simulink model "Crane_rigid_3d_single_20_coupling_tracking"  (R2021b)
settings: Solver=ode15s  StartTime=0.0  StopTime=t_f  MaxStep=1e-3  RelTol=1e-3
values from neighbouring files (symbols this model uses):
  h = 1e-5    (= 1e-05)    [Conference_paper.m]    (also in Latest.m)
  m = 10    [Conference_paper.m]    (also in Latest.m = 100; control_8_collocated_PD_tracking.m = load_mass+hook_mass+cable_mass_total)
  N = floor(t_f / h)    [control_2_zero_vibration.m]    (also in control_3_ZVD.m; modify_tracking.m = 3)
  s = c1*(x-xd)+c2*(v-vd)+c3*theta_dot_1+c4*theta_1    [control_10_SMC_single_first_explicit.m]    (also in control_11_SMC_single_first_implicit.m = c1*(x-xd)+c2*(v-vd)+c3*theta_dot+c4*theta; control_12_SMC_single_last_explicit.m = c1*(x-xd)+c2*(v-vd)+c3*theta_dot_2+c4*theta_2; control_13_SMC_single_last_implicit.m = c1*(x-xd)+c2*(v-vd)+c3*theta_dot+c4*theta; control_14_SMC_double_explicit.m = (v-vd)+lambda*(x-xd)+alpha*theta_1+beta*theta_2)
  sin_traj_w = 0.5    [modify_tracking.m]
  X = ex+lambda*sin(theta)    [control_16_PD_energy_first.m]    (also in control_17_PD_energy_last.m)
  Z = cont_param_8(4)    [control_8_collocated_PD_tracking.m]
undefined symbols (not defined in the file or in its folder): all_initial_sway, c_actuator, cable_mass_total, cart_disturbance_amp, cart_mass, delay_time, first_link_sway, hook_mass, load_disturbance_amp, payload_mass, sat_const, sin_traj_A, total_mass, traj_number, Y
libraries: nesl_utility x19, sm_lib x15
settings Model: Creator=rmoja  LastModifiedBy=SESA642626

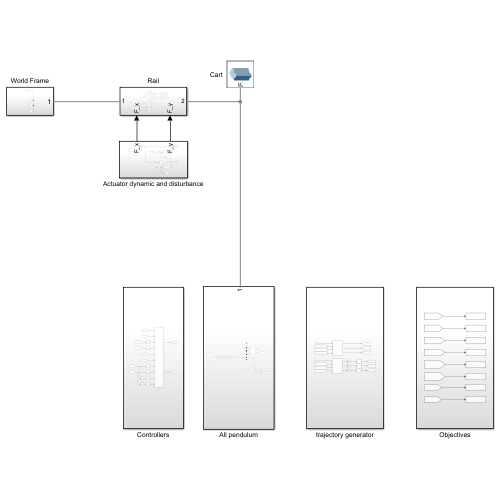
[thumbnail: Simulink's stored preview of the top-level diagram]
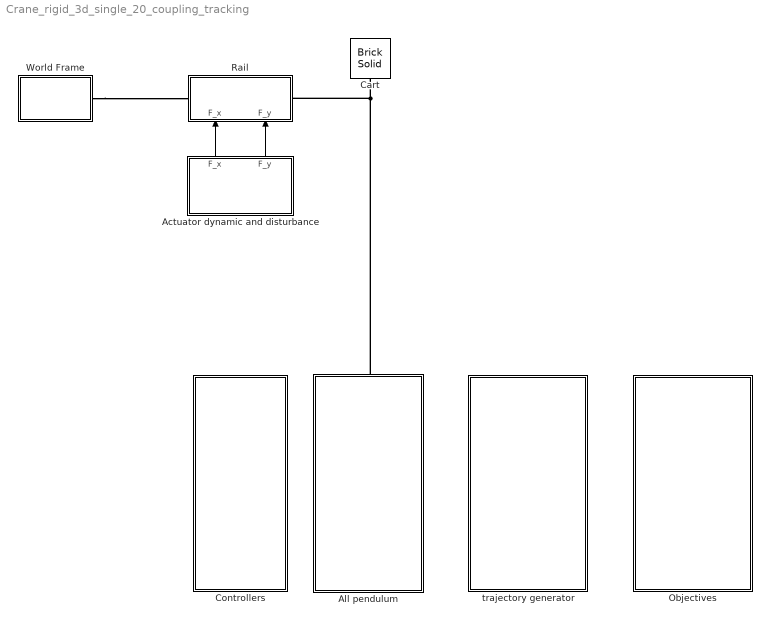
== system Crane_rigid_3d_single_20_coupling_tracking ==
  Actuator dynamic and disturbance : Subsystem
  All pendulum : Subsystem
      settings: PortSchema="{\"entries\":[{\"content\":{\"sides\":[{\"content\":{\"connectorIds\":[]},\"type\":\"ConnectorPlacement.EquallySpacedRectSide\",\"uuid\":\"a0695cec-8b60-4481-8da3-91054655feca\"},{\"content\":{\"connectorIds\":[],\"side\":\"RIGHT\"},\"type\":\"ConnectorPlacement.EquallySpacedRectSide\",\"uuid\":\"63fc90b5-61bb-43b2-b1de-87e85d16d1ba\"},{\"content\":{\"connectorIds\":[\"LConn1\"],\"side\":\"TOP\"},\"type\":\"ConnectorPlacement.EquallySpacedRectSide\",\"uuid\":\"b1a79959-5d9b-4237-a357-9ee6cf3ddb2d\"}]},\"type\":\"ConnectorPlacement.EquallySpacedConnector\",\"uuid\":\"2998d234-7b55-409a-8879-2241677dc568\"}],\"packageUris\":[\"http://schema.mathworks.com/mf0/Connector/R2020b\"],\"version\":\"1.0\"}"
  Cart : sm_lib/Body Elements/Brick Solid  GraphicAmbientColor=[0.15 0.15 0.15 1.0]  BasedOnType=Mass  BrickDimensions=[1 1 1]  BrickDimensionUnits=m  CenterOfMass=[0 0 0]  CenterOfMassUnits=m  GraphicDiffuseColor=[0.8 0.0 0.8]  Density=1000  DensityUnits=kg/(m^3)  DoExposeReferenceFrame=on  GraphicEmissiveColor=[0.0 0.0 0.0 1.0]  ExportEntireGeometry=off  SerializedFrames=<Frames/>  MarkerShape=Sphere  MarkerSize=10  GraphicType=FromGeometry  InertiaType=PointMass  Mass=cart_mass  MassUnits=kg  MomentsOfInertia=[1 1 1]  MomentsOfInertiaUnits=kg*m^2  GraphicOpacity=1.0  ProductsOfInertia=[0 0 0]  ProductsOfInertiaUnits=kg*m^2  GraphicShininess=75  GraphicSpecularColor=[0.5 0.5 0.5 1.0]  GraphicVisPropType=SimpleVisualProperties
  Controllers : Subsystem
  Objectives : Subsystem
  Rail : Subsystem
      settings: PortSchema="{\"entries\":[{\"content\":{\"sides\":[{\"content\":{\"connectorIds\":[\"LConn1\"]},\"type\":\"ConnectorPlacement.EquallySpacedRectSide\",\"uuid\":\"d9e65a69-c05e-4610-81fe-2f9f88514456\"},{\"content\":{\"connectorIds\":[\"RConn1\"],\"side\":\"RIGHT\"},\"type\":\"ConnectorPlacement.EquallySpacedRectSide\",\"uuid\":\"de9124b5-abd7-4a44-8ac0-9f1bb82b9c20\"},{\"content\":{\"connectorIds\":[],\"side\":\"TOP\"},\"type\":\"ConnectorPlacement.EquallySpacedRectSide\",\"uuid\":\"433c8926-32eb-4eac-9405-2f674875eeab\"},{\"content\":{\"connectorIds\":[\"In1\",\"In2\"],\"side\":\"BOTTOM\"},\"type\":\"ConnectorPlacement.EquallySpacedRectSide\",\"uuid\":\"d2188721-54bd-44ea-91c1-f694293db46f\"}]},\"type\":\"ConnectorPlacement.EquallySpacedConnector\",\"uuid\":\"441db2e5-934f-48d0-8bd6-b56c902c81c4\"}],\"packageUris\":[\"http://schema.mathworks.com/mf0/Connector/R2020b\"],\"version\":\"1.0\"}"
  World Frame : Subsystem
  trajectory generator : Subsystem
  wires:
  Actuator dynamic and disturbance/1(F_x) -> Rail/1(F_x)
  Actuator dynamic and disturbance/2(F_y) -> Rail/2(F_y)
  connections:
  World Frame/LConn1 -- Rail/LConn1
  All pendulum/LConn1 -- Rail/RConn1 -- Cart/RConn1

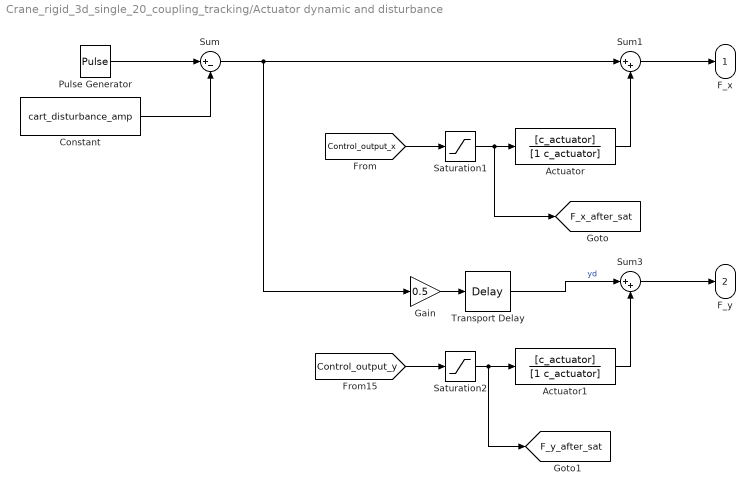
== system Crane_rigid_3d_single_20_coupling_tracking/Actuator dynamic and disturbance ==
  Actuator : TransferFcn  Numerator=[c_actuator]  Denominator=[1 c_actuator]
  Actuator1 : TransferFcn  Numerator=[c_actuator]  Denominator=[1 c_actuator]
  Constant : Constant  Value=cart_disturbance_amp
  Gain : Gain  Gain=0.5
  Pulse Generator : DiscretePulseGenerator  PulseType=Time based  Amplitude=2*cart_disturbance_amp  Period=20  PulseWidth=50
  Saturation1 : Saturate  UpperLimit=+sat_const  LowerLimit=-sat_const
  Saturation2 : Saturate  UpperLimit=+sat_const  LowerLimit=-sat_const
  Sum : Sum  Inputs=|+-
  Sum1 : Sum  Inputs=|++
  Sum3 : Sum  Inputs=|++
  Transport Delay : TransportDelay  BufferSize=8192
  F_x : Outport
  F_y : Outport  Port=2
  tag scope: F_x_after_sat=global, F_y_after_sat=global
  wires:
  Actuator/1 -> Sum1/2
  Sum1/1 -> F_x/1
  Saturation1/1 -> [F_x_after_sat], Actuator/1
  [Control_output_x] -> Saturation1/1
  Sum3/1 -> F_y/1
  [Control_output_y] -> Saturation2/1
  Saturation2/1 -> [F_y_after_sat], Actuator1/1
  Actuator1/1 -> Sum3/2
  Pulse Generator/1 -> Sum/1
  Constant/1 -> Sum/2
  Sum/1 -> Gain/1, Sum1/1
  Gain/1 -> Transport Delay/1
  Transport Delay/1 -> Sum3/1  "yd"

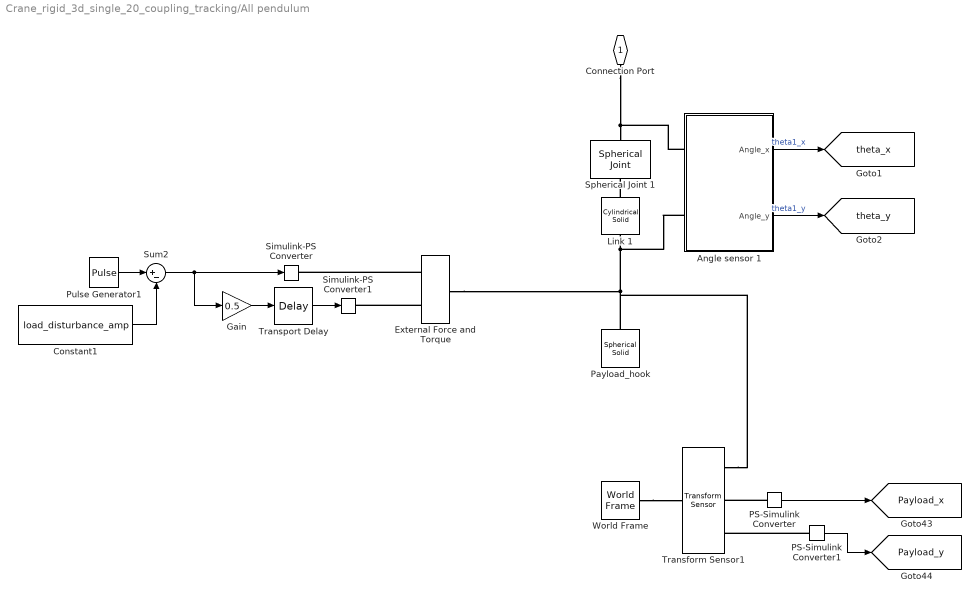
== system Crane_rigid_3d_single_20_coupling_tracking/All pendulum ==
  Angle sensor 1 : Subsystem
  Constant1 : Constant  Value=load_disturbance_amp
  External Force and Torque : sm_lib/Forces and Torques/External Force and Torque  ForceResolutionFrame=World  EnableForceX=on  EnableForceY=on  EnableForceZ=off  EnableForce=off  TorqueResolutionFrame=AttachedFrame  EnableTorqueX=off  EnableTorqueY=off  EnableTorqueZ=off  EnableTorque=off
  Gain : Gain  Gain=0.5
  Link 1 : sm_lib/Body Elements/Cylindrical Solid  GraphicAmbientColor=[0.15 0.15 0.15 1.0]  BasedOnType=Mass  CenterOfMass=[0 0 0]  CenterOfMassUnits=m  GraphicDiffuseColor=[0.5 0.5 0.5]  CylinderLength=cable_length  CylinderLengthUnits=m  CylinderRadius=0.02  CylinderRadiusUnits=m  Density=1000  DensityUnits=kg/m^3  DoExposeReferenceFrame=off  GraphicEmissiveColor=[0.0 0.0 0.0 1.0]  ExportEntireGeometry=off  SerializedFrames=<Frames><Frame><Id>Frame1</Id><Value><Name>F1</Name><Origin><Source>GeometricFeature</Source><FeatureName>top surface</FeatureName></Origin><PrimaryAxis><DefinedDirection>+Z</DefinedDirection><Source>ReferenceFrame</Source><SourceDirection>+Z</SourceDirection><FeatureName></FeatureName></PrimaryAxis><SecondaryAxis><DefinedDirection>+X</DefinedDirection><Source>ReferenceFrame</Source><SourceDirection>+X</SourceDirection><FeatureName></FeatureName></SecondaryAxis></Value></Frame><Frame><Id>Frame2</Id><Value><Name>F2</Name><Origin><Source>GeometricFeature</Source><FeatureName>bottom curve</FeatureName></Origin><PrimaryAxis><DefinedDirection>+Z</DefinedDirection><Source>ReferenceFrame</Source><SourceDirection>+Z</SourceDirection><FeatureName></FeatureName></PrimaryAxis><SecondaryAxis><DefinedDirection>+X</DefinedDirection><Source>ReferenceFrame</Source><SourceDirection>+X</SourceDirection><FeatureName></FeatureName></SecondaryAxis></Value></Frame></Frames>  MarkerShape=Sphere  MarkerSize=10  GraphicType=FromGeometry  InertiaType=CalculateFromGeometry  Mass=cable_mass_total  MassUnits=kg  MomentsOfInertia=[1 1 1]  MomentsOfInertiaUnits=kg*m^2  GraphicOpacity=1.0  ProductsOfInertia=[0 0 0]  ProductsOfInertiaUnits=kg*m^2  GraphicShininess=75  GraphicSpecularColor=[0.5 0.5 0.5 1.0]  GraphicVisPropType=SimpleVisualProperties
  PS-Simulink Converter : nesl_utility/PS-Simulink Converter  PhysicalDomain=network_engine_domain  SubClassName=ps_output  LeftPortType=input  RightPortType=output  PseudoPeriodic=off  Frequencies=[]  Unit=inherit  AffineConversion=off
      settings: SourceProductBaseCode=PW,SS
  PS-Simulink Converter1 : nesl_utility/PS-Simulink Converter  PhysicalDomain=network_engine_domain  SubClassName=ps_output  LeftPortType=input  RightPortType=output  PseudoPeriodic=off  Frequencies=[]  Unit=inherit  AffineConversion=off
      settings: SourceProductBaseCode=PW,SS
  Payload_hook : sm_lib/Body Elements/Spherical Solid  GraphicAmbientColor=[0.15 0.15 0.15 1.0]  BasedOnType=Density  CenterOfMass=[0 0 0]  CenterOfMassUnits=m  GraphicDiffuseColor=[1.0 0.2 0.0]  Density=1000  DensityUnits=kg/(m^3)  DoExposeReferenceFrame=on  GraphicEmissiveColor=[0.0 0.0 0.0 1.0]  ExportEntireGeometry=off  SerializedExposedGeometries=<ExposedGeometries/>  SerializedFrames=<Frames/>  MarkerShape=Sphere  MarkerSize=10  GraphicType=FromGeometry  InertiaType=PointMass  Mass=payload_mass+hook_mass  MassUnits=kg  MomentsOfInertia=[1 1 1]*1e-3  MomentsOfInertiaUnits=kg*m^2  GraphicOpacity=1.0  ProductsOfInertia=[0 0 0]  ProductsOfInertiaUnits=kg*m^2  GraphicShininess=75  GraphicSpecularColor=[0.5 0.5 0.5 1.0]  SphereRadius=0.05  SphereRadiusUnits=m  GraphicVisPropType=SimpleVisualProperties
  Pulse Generator1 : DiscretePulseGenerator  PulseType=Time based  Amplitude=2*load_disturbance_amp  Period=20  PulseWidth=50
  Simulink-PS Converter : nesl_utility/Simulink-PS Converter  PhysicalDomain=network_engine_domain  SubClassName=ps_input  LeftPortType=input  RightPortType=output  PseudoPeriodic=off  Frequencies=[]  NoiseDistribution=none  NoiseParameters=[]  Unit=1  AffineConversion=off  FilteringAndDerivatives=provide  SimscapeFilterOrder=1  InputFilterTimeConstant=0.001  UdotUserProvided=0
      settings: SourceProductBaseCode=PW,SS
  Simulink-PS Converter1 : nesl_utility/Simulink-PS Converter  PhysicalDomain=network_engine_domain  SubClassName=ps_input  LeftPortType=input  RightPortType=output  PseudoPeriodic=off  Frequencies=[]  NoiseDistribution=none  NoiseParameters=[]  Unit=1  AffineConversion=off  FilteringAndDerivatives=provide  SimscapeFilterOrder=1  InputFilterTimeConstant=0.001  UdotUserProvided=0
      settings: SourceProductBaseCode=PW,SS
  Spherical Joint 1 : sm_lib/Joints/Spherical Joint  JointMode=Normal  SenseConstraintForce=off  SenseConstraintForceX=off  SenseConstraintForceY=off  SenseConstraintForceZ=off  SenseConstraintTorque=off  SenseConstraintTorqueX=off  SenseConstraintTorqueY=off  SenseConstraintTorqueZ=off  SenseTotalForce=off  SenseTotalForceX=off  SenseTotalForceY=off  SenseTotalForceZ=off  SenseTotalTorque=off  SenseTotalTorqueX=off  SenseTotalTorqueY=off  SenseTotalTorqueZ=off  CompositeWrenchDir=FollowerOnBase  CompositeWrenchFrame=BaseFrame  DefPosRotationMethod=None  DefPosRotationAngleUnits=deg  DefPosRotationStandardAxis=+Z  DefPosRotationAngle=0.0  DefPosRotationArbitraryAxis=[0 0 1]  DefPosFollAlignAxisA=+X  DefPosBaseAlignAxisA=+Y  DefPosFollAlignAxisB=+Y  DefPosBaseAlignAxisB=+Z  DefPosRotationSequenceAxes=FollowerAxes  DefPosRotationSequence=XYX  DefPosRotationSequenceAngles=[0 0 0]  DefPosRotationSequenceAnglesUnits=deg  DefPosRotationMatrix=[1 0 0; 0 1 0; 0 0 1]  EqPosRotationMethod=None  EqPosRotationAngleUnits=deg  EqPosRotationStandardAxis=+Z  EqPosRotationAngle=0.0  EqPosRotationArbitraryAxis=[0 0 1]  EqPosFollAlignAxisA=+X  EqPosBaseAlignAxisA=+Y  EqPosFollAlignAxisB=+Y  EqPosBaseAlignAxisB=+Z  EqPosRotationSequenceAxes=FollowerAxes  EqPosRotationSequence=XYX  EqPosRotationSequenceAngles=[0 0 0]  EqPosRotationSequenceAnglesUnits=deg  EqPosRotationMatrix=[1 0 0; 0 1 0; 0 0 1]  SpringStiffness=joint_stiffness  SpringStiffnessUnits=N*m/deg  DampingCoefficient=damping_coefficient  DampingCoefficientUnits=N*m/(deg/s)  ActuateTorqueX=off  ActuateTorqueY=off  ActuateTorqueZ=off  ActuateTorque=off  TorqueActuationMode=NoTorque  MotionActuationMode=ComputedMotion  ActuationFrame=BaseFrame  SensePosition=off  SenseVelocityX=off  SenseVelocityY=off  SenseVelocityZ=off  SenseVelocity=off  SenseAccelerationX=off  SenseAccelerationY=off  SenseAccelerationZ=off  SenseAcceleration=off  SenseTorqueX=off  SenseTorqueY=off  SenseTorqueZ=off  SenseTorqueForce=off  SenseLowerLimitTorqueMag=off  SenseUpperLimitTorqueMag=off  SensingFrame=BaseFrame  LowerLimitSpecify=off  LowerLimitBound=15  LowerLimitBoundUnits=deg  LowerLimitStiffness=1e4  LowerLimitStiffnessUnits=N*m/deg  LowerLimitDamping=10  LowerLimitDampingUnits=N*m/(deg/s)  LowerLimitTransitionRegionWidth=0.1  LowerLimitTransitionRegionWidthUnits=deg  UpperLimitSpecify=off  UpperLimitBound=45  UpperLimitBoundUnits=deg  UpperLimitStiffness=1e4  UpperLimitStiffnessUnits=N*m/deg  UpperLimitDamping=10  UpperLimitDampingUnits=N*m/(deg/s)  UpperLimitTransitionRegionWidth=0.1  UpperLimitTransitionRegionWidthUnits=deg  PositionTargetRotationMethod=StandardAxis  PositionTargetRotationAngleUnits=deg  PositionTargetRotationStandardAxis=+Y  PositionTargetRotationAngle=first_link_sway+all_initial_sway  PositionTargetRotationArbitraryAxis=[1 1 1]  PositionTargetFollAlignAxisA=+X  PositionTargetBaseAlignAxisA=-Z  PositionTargetFollAlignAxisB=+Y  PositionTargetBaseAlignAxisB=-Z  PositionTargetRotationSequenceAxes=BaseAxes  PositionTargetRotationSequence=XYX  PositionTargetRotationSequenceAngles=[15 0 0]  PositionTargetRotationSequenceAnglesUnits=deg  PositionTargetRotationMatrix=[1 0 0; 0 1 0; 0 0 1]  PositionTargetSpecify=on  PositionTargetPriority=High  VelocityTargetValue=[0 0 0]  VelocityTargetValueUnits=deg/s  VelocityTargetSpecify=off  VelocityTargetPriority=High  VelocityTargetInFollowerFrame=on
  Sum2 : Sum  Inputs=|+-
  Transform Sensor1 : sm_lib/Frames and Transforms/Transform Sensor  MeasurementFrame=World  SenseAngle=off  SenseAxis=off  SenseAngle1=off  SenseAngle2=off  SenseAngle3=off  SenseQ=off  SenseR=off  SenseOmegaX=off  SenseOmegaY=off  SenseOmegaZ=off  SenseOmega1=off  SenseOmega2=off  SenseOmega3=off  SenseQDot=off  SenseRDot=off  SenseAlphaX=off  SenseAlphaY=off  SenseAlphaZ=off  SenseAlpha1=off  SenseAlpha2=off  SenseAlpha3=off  SenseQDDot=off  SenseRDDot=off  SenseX=on  SenseY=on  SenseZ=off  SenseRad=off  SenseAzim=off  SenseDist=off  SenseInc=off  SenseXDot=off  SenseYDot=off  SenseZDot=off  SenseRadDot=off  SenseAzimDot=off  SenseDistDot=off  SenseIncDot=off  SenseXDDot=off  SenseYDDot=off  SenseZDDot=off  SenseRadDDot=off  SenseAzimDDot=off  SenseDistDDot=off  SenseIncDDot=off
  Transport Delay : TransportDelay  BufferSize=8192
  World Frame : sm_lib/Frames and Transforms/World Frame
  Connection Port : PMIOPort  Side=Left
  tag scope: Payload_x=global, Payload_y=global, theta_x=global, theta_y=global
  wires:
  Angle sensor 1/1(Angle_x) -> [theta_x]  "theta1_x"
  Angle sensor 1/2(Angle_y) -> [theta_y]  "theta1_y"
  Constant1/1 -> Sum2/2
  Pulse Generator1/1 -> Sum2/1
  Sum2/1 -> Gain/1, Simulink-PS Converter/1
  Gain/1 -> Transport Delay/1
  Transport Delay/1 -> Simulink-PS Converter1/1
  PS-Simulink Converter/1 -> [Payload_x]
  PS-Simulink Converter1/1 -> [Payload_y]
  connections:
  Angle sensor 1/LConn2 -- Transform Sensor1/RConn1 -- Payload_hook/RConn1 -- External Force and Torque/RConn1 -- Link 1/RConn1
  Connection Port/RConn1 -- Angle sensor 1/LConn1 -- Spherical Joint 1/LConn1
  Link 1/LConn1 -- Spherical Joint 1/RConn1
  External Force and Torque/LConn1 -- Simulink-PS Converter/RConn1
  External Force and Torque/LConn2 -- Simulink-PS Converter1/RConn1
  PS-Simulink Converter1/LConn1 -- Transform Sensor1/RConn3
  World Frame/RConn1 -- Transform Sensor1/LConn1
  PS-Simulink Converter/LConn1 -- Transform Sensor1/RConn2

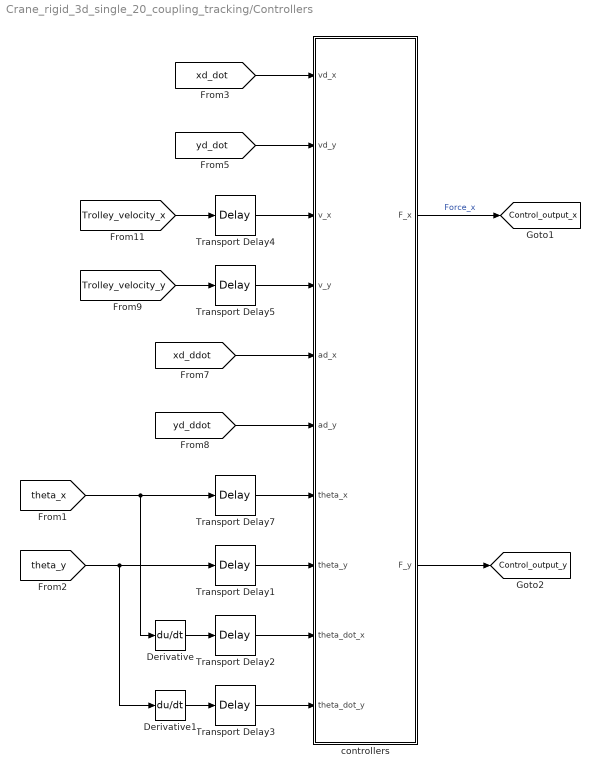
== system Crane_rigid_3d_single_20_coupling_tracking/Controllers ==
  Derivative : Derivative
  Derivative1 : Derivative
  Transport Delay{1..5,7} (6 alike) : TransportDelay  DelayTime=delay_time  BufferSize=8192
  controllers : Subsystem  TreatAsAtomicUnit=on  SystemSampleTime=h
  tag scope: Control_output_x=global, Control_output_y=global
  wires:
  [theta_x] -> Derivative/1, Transport Delay7/1
  Transport Delay7/1 -> controllers/7(theta_x)
  controllers/1(F_x) -> [Control_output_x]  "Force_x"
  controllers/2(F_y) -> [Control_output_y]
  Transport Delay1/1 -> controllers/8(theta_y)
  [theta_y] -> Derivative1/1, Transport Delay1/1
  Transport Delay2/1 -> controllers/9(theta_dot_x)
  Transport Delay3/1 -> controllers/10(theta_dot_y)
  Derivative/1 -> Transport Delay2/1
  Derivative1/1 -> Transport Delay3/1
  [xd_dot] -> controllers/1(vd_x)
  [yd_dot] -> controllers/2(vd_y)
  [Trolley_velocity_x] -> Transport Delay4/1
  Transport Delay4/1 -> controllers/3(v_x)
  [Trolley_velocity_y] -> Transport Delay5/1
  Transport Delay5/1 -> controllers/4(v_y)
  [xd_ddot] -> controllers/5(ad_x)
  [yd_ddot] -> controllers/6(ad_y)

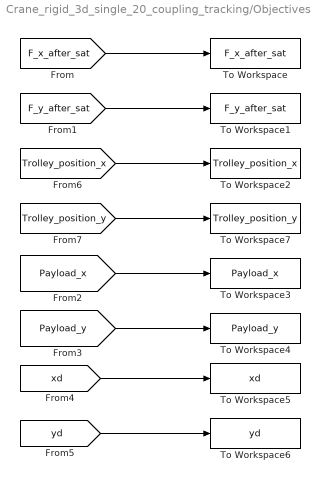
== system Crane_rigid_3d_single_20_coupling_tracking/Objectives ==
  To Workspace : ToWorkspace  VariableName=F_x_after_sat  SampleTime=h
  To Workspace1 : ToWorkspace  VariableName=F_y_after_sat  SampleTime=h
  To Workspace2 : ToWorkspace  VariableName=Trolley_position_x  SampleTime=h
  To Workspace3 : ToWorkspace  VariableName=Payload_x  SampleTime=h
  To Workspace4 : ToWorkspace  VariableName=Payload_y  SampleTime=h
  To Workspace5 : ToWorkspace  VariableName=xd  SampleTime=h
  To Workspace6 : ToWorkspace  VariableName=yd  SampleTime=h
  To Workspace7 : ToWorkspace  VariableName=Trolley_position_y  SampleTime=h
  wires:
  [F_x_after_sat] -> To Workspace/1
  [F_y_after_sat] -> To Workspace1/1
  [Trolley_position_x] -> To Workspace2/1
  [Payload_x] -> To Workspace3/1
  [Payload_y] -> To Workspace4/1
  [xd] -> To Workspace5/1
  [yd] -> To Workspace6/1
  [Trolley_position_y] -> To Workspace7/1

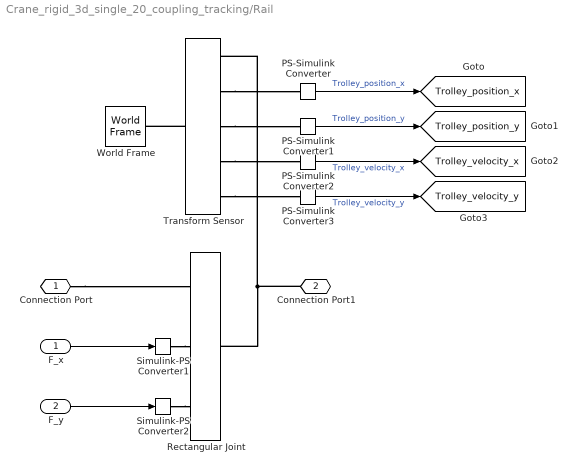
== system Crane_rigid_3d_single_20_coupling_tracking/Rail ==
  F_x : Inport
  F_y : Inport  Port=2
  PS-Simulink Converter{,1..3} (4 alike) : nesl_utility/PS-Simulink Converter  PhysicalDomain=network_engine_domain  SubClassName=ps_output  LeftPortType=input  RightPortType=output  PseudoPeriodic=off  Frequencies=[]  Unit=inherit  AffineConversion=off
      settings: SourceProductBaseCode=PW,SS
  Rectangular Joint : sm_lib/Joints/Rectangular Joint  JointMode=Normal  SenseConstraintForce=off  SenseConstraintForceX=off  SenseConstraintForceY=off  SenseConstraintForceZ=off  SenseConstraintTorque=off  SenseConstraintTorqueX=off  SenseConstraintTorqueY=off  SenseConstraintTorqueZ=off  SenseTotalForce=off  SenseTotalForceX=off  SenseTotalForceY=off  SenseTotalForceZ=off  SenseTotalTorque=off  SenseTotalTorqueX=off  SenseTotalTorqueY=off  SenseTotalTorqueZ=off  CompositeWrenchDir=FollowerOnBase  CompositeWrenchFrame=BaseFrame  PxEquilibriumPosition=0  PxEquilibriumPositionUnits=m  PxSpringStiffness=0  PxSpringStiffnessUnits=N/m  PxDampingCoefficient=0  PxDampingCoefficientUnits=N/(m/s)  PxTorqueActuationMode=InputTorque  PxMotionActuationMode=ComputedMotion  PxSensePosition=off  PxSenseVelocity=off  PxSenseAcceleration=off  PxSenseTorqueForce=off  PxSenseLowerLimitTorqueForce=off  PxSenseUpperLimitTorqueForce=off  PxLowerLimitSpecify=off  PxLowerLimitBound=-1  PxLowerLimitBoundUnits=m  PxLowerLimitStiffness=1e6  PxLowerLimitStiffnessUnits=N/m  PxLowerLimitDamping=1e3  PxLowerLimitDampingUnits=N/(m/s)  PxLowerLimitTransitionRegionWidth=1e-4  PxLowerLimitTransitionRegionWidthUnits=m  PxUpperLimitSpecify=off  PxUpperLimitBound=1  PxUpperLimitBoundUnits=m  PxUpperLimitStiffness=1e6  PxUpperLimitStiffnessUnits=N/m  PxUpperLimitDamping=1e3  PxUpperLimitDampingUnits=N/(m/s)  PxUpperLimitTransitionRegionWidth=1e-4  PxUpperLimitTransitionRegionWidthUnits=m  PxPositionTargetSpecify=off  PxPositionTargetPriority=High  PxPositionTargetValue=0  PxPositionTargetValueUnits=m  PxVelocityTargetSpecify=off  PxVelocityTargetPriority=High  PxVelocityTargetValue=0  PxVelocityTargetValueUnits=m/s  PyEquilibriumPosition=0  PyEquilibriumPositionUnits=m  PySpringStiffness=0  PySpringStiffnessUnits=N/m  PyDampingCoefficient=0  PyDampingCoefficientUnits=N/(m/s)  PyTorqueActuationMode=InputTorque  PyMotionActuationMode=ComputedMotion  PySensePosition=off  PySenseVelocity=off  PySenseAcceleration=off  PySenseTorqueForce=off  PySenseLowerLimitTorqueForce=off  PySenseUpperLimitTorqueForce=off  PyLowerLimitSpecify=off  PyLowerLimitBound=-1  PyLowerLimitBoundUnits=m  PyLowerLimitStiffness=1e6  PyLowerLimitStiffnessUnits=N/m  PyLowerLimitDamping=1e3  PyLowerLimitDampingUnits=N/(m/s)  PyLowerLimitTransitionRegionWidth=1e-4  PyLowerLimitTransitionRegionWidthUnits=m  PyUpperLimitSpecify=off  PyUpperLimitBound=1  PyUpperLimitBoundUnits=m  PyUpperLimitStiffness=1e6  PyUpperLimitStiffnessUnits=N/m  PyUpperLimitDamping=1e3  PyUpperLimitDampingUnits=N/(m/s)  PyUpperLimitTransitionRegionWidth=1e-4  PyUpperLimitTransitionRegionWidthUnits=m  PyPositionTargetSpecify=off  PyPositionTargetPriority=High  PyPositionTargetValue=0  PyPositionTargetValueUnits=m  PyVelocityTargetSpecify=off  PyVelocityTargetPriority=High  PyVelocityTargetValue=0  PyVelocityTargetValueUnits=m/s
  Simulink-PS Converter1 : nesl_utility/Simulink-PS Converter  PhysicalDomain=network_engine_domain  SubClassName=ps_input  LeftPortType=input  RightPortType=output  PseudoPeriodic=off  Frequencies=[]  NoiseDistribution=none  NoiseParameters=[]  Unit=1  AffineConversion=off  FilteringAndDerivatives=provide  SimscapeFilterOrder=1  InputFilterTimeConstant=0.001  UdotUserProvided=0
      settings: SourceProductBaseCode=PW,SS
  Simulink-PS Converter2 : nesl_utility/Simulink-PS Converter  PhysicalDomain=network_engine_domain  SubClassName=ps_input  LeftPortType=input  RightPortType=output  PseudoPeriodic=off  Frequencies=[]  NoiseDistribution=none  NoiseParameters=[]  Unit=1  AffineConversion=off  FilteringAndDerivatives=provide  SimscapeFilterOrder=1  InputFilterTimeConstant=0.001  UdotUserProvided=0
      settings: SourceProductBaseCode=PW,SS
  Transform Sensor : sm_lib/Frames and Transforms/Transform Sensor  MeasurementFrame=World  SenseAngle=off  SenseAxis=off  SenseAngle1=off  SenseAngle2=off  SenseAngle3=off  SenseQ=off  SenseR=off  SenseOmegaX=off  SenseOmegaY=off  SenseOmegaZ=off  SenseOmega1=off  SenseOmega2=off  SenseOmega3=off  SenseQDot=off  SenseRDot=off  SenseAlphaX=off  SenseAlphaY=off  SenseAlphaZ=off  SenseAlpha1=off  SenseAlpha2=off  SenseAlpha3=off  SenseQDDot=off  SenseRDDot=off  SenseX=on  SenseY=on  SenseZ=off  SenseRad=off  SenseAzim=off  SenseDist=off  SenseInc=off  SenseXDot=on  SenseYDot=on  SenseZDot=off  SenseRadDot=off  SenseAzimDot=off  SenseDistDot=off  SenseIncDot=off  SenseXDDot=off  SenseYDDot=off  SenseZDDot=off  SenseRadDDot=off  SenseAzimDDot=off  SenseDistDDot=off  SenseIncDDot=off
  World Frame : sm_lib/Frames and Transforms/World Frame
  Connection Port : PMIOPort  Side=Left
  Connection Port1 : PMIOPort  Port=2  Side=Right
  tag scope: Trolley_position_x=global, Trolley_position_y=global, Trolley_velocity_x=global, Trolley_velocity_y=global
  wires:
  PS-Simulink Converter/1 -> [Trolley_position_x]  "Trolley_position_x"
  PS-Simulink Converter1/1 -> [Trolley_position_y]  "Trolley_position_y"
  PS-Simulink Converter2/1 -> [Trolley_velocity_x]  "Trolley_velocity_x"
  PS-Simulink Converter3/1 -> [Trolley_velocity_y]  "Trolley_velocity_y"
  F_x/1 -> Simulink-PS Converter1/1
  F_y/1 -> Simulink-PS Converter2/1
  connections:
  Connection Port/RConn1 -- Rectangular Joint/LConn1
  Connection Port1/RConn1 -- Rectangular Joint/RConn1 -- Transform Sensor/RConn1
  Transform Sensor/LConn1 -- World Frame/RConn1
  Transform Sensor/RConn2 -- PS-Simulink Converter/LConn1
  Transform Sensor/RConn3 -- PS-Simulink Converter1/LConn1
  Transform Sensor/RConn4 -- PS-Simulink Converter2/LConn1
  Transform Sensor/RConn5 -- PS-Simulink Converter3/LConn1
  Simulink-PS Converter1/RConn1 -- Rectangular Joint/LConn2
  Simulink-PS Converter2/RConn1 -- Rectangular Joint/LConn3

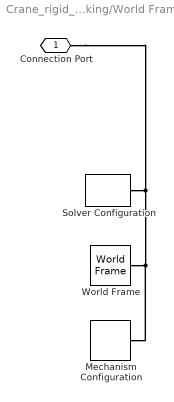
== system Crane_rigid_3d_single_20_coupling_tracking/World Frame ==
  Mechanism Configuration : sm_lib/Utilities/Mechanism Configuration  UniformGravity=Constant  GravityVector=[0 0 -9.80665]  GravityUnits=m/s^2  LinearizationDelta=0.001  JointModeTransitionNonlinearIterations=2
  Solver Configuration : nesl_utility/Solver Configuration  PhysicalDomain=network_engine_domain  SubClassName=solver  LeftPortType=input  RightPortType=generic  Tones=[]  Harmonics=[]  SimulateNoise=off  Profile=off  UseLocalSampling=off  EnableSwitchedLinearOptims=on  FrequencyDomain=off  UseCCode=off  RelTol=0.001  AbsTol=1e-06  MinStep=1e-09  ToWorkspace=off  RevertToSquareIcSolve=off  NumHomotopyIterations=100  PhasorMode=off  PhasorModeNumHarmonics=1  DoDC=off  ResidualTolerance=1e-09  UseLocalSolver=off  LocalSolverChoice=NE_BACKWARD_EULER_ADVANCER  LocalSolverSampleTime=0.001  DoFixedCost=off  MaxNonlinIter=3  MaxModeIter=2  ComputeImpulses=off  ImpulseIterations=2  LinearAlgebra=auto  EquationFormulation=NE_TIME_EF  DelaysMemoryBudget=1024  AutomaticFiltering=on  FilteringTimeConstant=0.001  PartitionStorageMethod=AS_NEEDED  PartitionMemoryBudget=1024  PartitionMethod=ROBUST
      settings: SourceProductBaseCode=PW,SS
  World Frame : sm_lib/Frames and Transforms/World Frame
  Connection Port : PMIOPort  Side=Left
  connections:
  Solver Configuration/RConn1 -- Connection Port/RConn1 -- Mechanism Configuration/RConn1 -- World Frame/RConn1

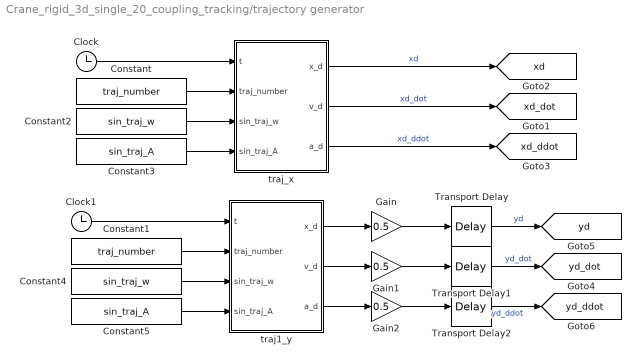
== system Crane_rigid_3d_single_20_coupling_tracking/trajectory generator ==
  Clock : Clock
  Clock1 : Clock
  Constant : Constant  Value=traj_number
  Constant1 : Constant  Value=traj_number
  Constant2 : Constant  Value=sin_traj_w
  Constant3 : Constant  Value=sin_traj_A
  Constant4 : Constant  Value=sin_traj_w
  Constant5 : Constant  Value=sin_traj_A
  Gain : Gain  Gain=0.5
  Gain1 : Gain  Gain=0.5
  Gain2 : Gain  Gain=0.5
  Transport Delay : TransportDelay  BufferSize=8192
  Transport Delay1 : TransportDelay  BufferSize=8192
  Transport Delay2 : TransportDelay  BufferSize=8192
  traj1_y : MATLAB Function  TreatAsAtomicUnit=on
  traj_x : MATLAB Function  TreatAsAtomicUnit=on
  tag scope: xd=global, xd_ddot=global, xd_dot=global, yd=global, yd_ddot=global, yd_dot=global
  wires:
  traj_x/1(x_d) -> [xd]  "xd"
  Clock/1 -> traj_x/1(t)
  traj_x/2(v_d) -> [xd_dot]  "xd_dot"
  traj_x/3(a_d) -> [xd_ddot]  "xd_ddot"
  Constant/1 -> traj_x/2(traj_number)
  traj1_y/3(a_d) -> Gain2/1
  traj1_y/2(v_d) -> Gain1/1
  traj1_y/1(x_d) -> Gain/1
  Gain/1 -> Transport Delay/1
  Transport Delay/1 -> [yd]  "yd"
  Gain1/1 -> Transport Delay1/1
  Transport Delay1/1 -> [yd_dot]  "yd_dot"
  Gain2/1 -> Transport Delay2/1
  Transport Delay2/1 -> [yd_ddot]  "yd_ddot"
  Constant2/1 -> traj_x/3(sin_traj_w)
  Constant3/1 -> traj_x/4(sin_traj_A)
  Constant5/1 -> traj1_y/4(sin_traj_A)
  Constant4/1 -> traj1_y/3(sin_traj_w)
  Constant1/1 -> traj1_y/2(traj_number)
  Clock1/1 -> traj1_y/1(t)

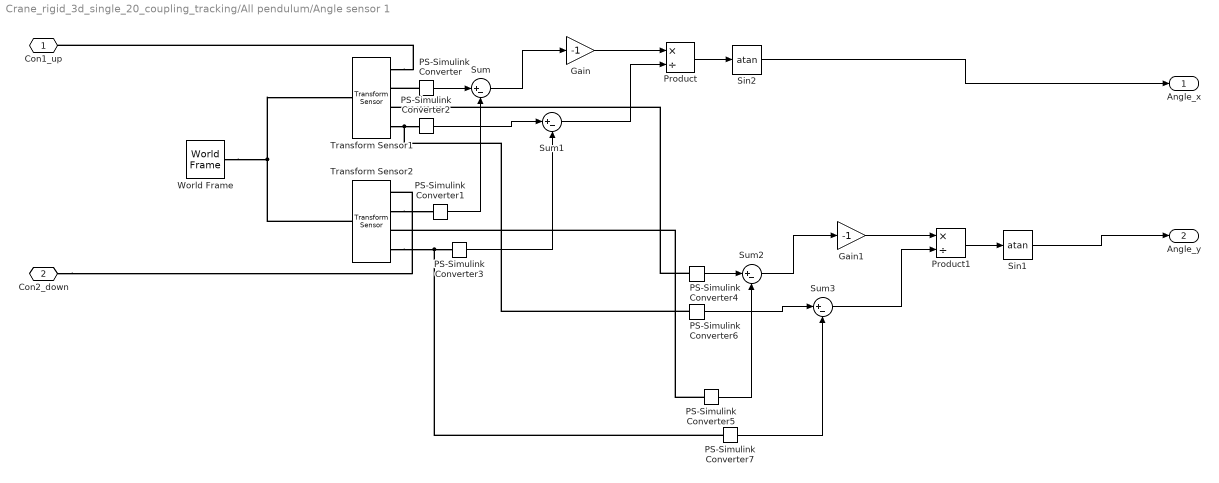
== system Crane_rigid_3d_single_20_coupling_tracking/All pendulum/Angle sensor 1 ==
  Gain : Gain  Gain=-1
  Gain1 : Gain  Gain=-1
  PS-Simulink Converter{,1..7} (8 alike) : nesl_utility/PS-Simulink Converter  PhysicalDomain=network_engine_domain  SubClassName=ps_output  LeftPortType=input  RightPortType=output  PseudoPeriodic=off  Frequencies=[]  Unit=inherit  AffineConversion=off
      settings: SourceProductBaseCode=PW,SS
  Product : Product  Inputs=*/
  Product1 : Product  Inputs=*/
  Sin1 : Trigonometry  Operator=atan
  Sin2 : Trigonometry  Operator=atan
  Sum{,1..3} (4 alike) : Sum  Inputs=|+-
  Transform Sensor1 : sm_lib/Frames and Transforms/Transform Sensor  MeasurementFrame=World  SenseAngle=off  SenseAxis=off  SenseAngle1=off  SenseAngle2=off  SenseAngle3=off  SenseQ=off  SenseR=off  SenseOmegaX=off  SenseOmegaY=off  SenseOmegaZ=off  SenseOmega1=off  SenseOmega2=off  SenseOmega3=off  SenseQDot=off  SenseRDot=off  SenseAlphaX=off  SenseAlphaY=off  SenseAlphaZ=off  SenseAlpha1=off  SenseAlpha2=off  SenseAlpha3=off  SenseQDDot=off  SenseRDDot=off  SenseX=on  SenseY=on  SenseZ=on  SenseRad=off  SenseAzim=off  SenseDist=off  SenseInc=off  SenseXDot=off  SenseYDot=off  SenseZDot=off  SenseRadDot=off  SenseAzimDot=off  SenseDistDot=off  SenseIncDot=off  SenseXDDot=off  SenseYDDot=off  SenseZDDot=off  SenseRadDDot=off  SenseAzimDDot=off  SenseDistDDot=off  SenseIncDDot=off
  Transform Sensor2 : sm_lib/Frames and Transforms/Transform Sensor  MeasurementFrame=World  SenseAngle=off  SenseAxis=off  SenseAngle1=off  SenseAngle2=off  SenseAngle3=off  SenseQ=off  SenseR=off  SenseOmegaX=off  SenseOmegaY=off  SenseOmegaZ=off  SenseOmega1=off  SenseOmega2=off  SenseOmega3=off  SenseQDot=off  SenseRDot=off  SenseAlphaX=off  SenseAlphaY=off  SenseAlphaZ=off  SenseAlpha1=off  SenseAlpha2=off  SenseAlpha3=off  SenseQDDot=off  SenseRDDot=off  SenseX=on  SenseY=on  SenseZ=on  SenseRad=off  SenseAzim=off  SenseDist=off  SenseInc=off  SenseXDot=off  SenseYDot=off  SenseZDot=off  SenseRadDot=off  SenseAzimDot=off  SenseDistDot=off  SenseIncDot=off  SenseXDDot=off  SenseYDDot=off  SenseZDDot=off  SenseRadDDot=off  SenseAzimDDot=off  SenseDistDDot=off  SenseIncDDot=off
  World Frame : sm_lib/Frames and Transforms/World Frame
  Con1_up : PMIOPort  Side=Left
  Con2_down : PMIOPort  Port=2  Side=Left
  Angle_x : Outport
  Angle_y : Outport  Port=2
  wires:
  PS-Simulink Converter/1 -> Sum/1
  Sum1/1 -> Product/2
  Product/1 -> Sin2/1
  PS-Simulink Converter2/1 -> Sum1/1
  PS-Simulink Converter3/1 -> Sum1/2
  Gain/1 -> Product/1
  PS-Simulink Converter7/1 -> Sum3/2
  PS-Simulink Converter4/1 -> Sum2/1
  PS-Simulink Converter5/1 -> Sum2/2
  PS-Simulink Converter1/1 -> Sum/2
  PS-Simulink Converter6/1 -> Sum3/1
  Product1/1 -> Sin1/1
  Sum2/1 -> Gain1/1
  Sum3/1 -> Product1/2
  Gain1/1 -> Product1/1
  Sum/1 -> Gain/1
  Sin2/1 -> Angle_x/1
  Sin1/1 -> Angle_y/1
  connections:
  World Frame/RConn1 -- Transform Sensor2/LConn1 -- Transform Sensor1/LConn1
  Transform Sensor2/RConn4 -- PS-Simulink Converter7/LConn1 -- PS-Simulink Converter3/LConn1
  Transform Sensor1/RConn4 -- PS-Simulink Converter6/LConn1 -- PS-Simulink Converter2/LConn1
  PS-Simulink Converter5/LConn1 -- Transform Sensor2/RConn3
  PS-Simulink Converter4/LConn1 -- Transform Sensor1/RConn3
  Transform Sensor2/RConn2 -- PS-Simulink Converter1/LConn1
  PS-Simulink Converter/LConn1 -- Transform Sensor1/RConn2
  Transform Sensor1/RConn1 -- Con1_up/RConn1
  Con2_down/RConn1 -- Transform Sensor2/RConn1

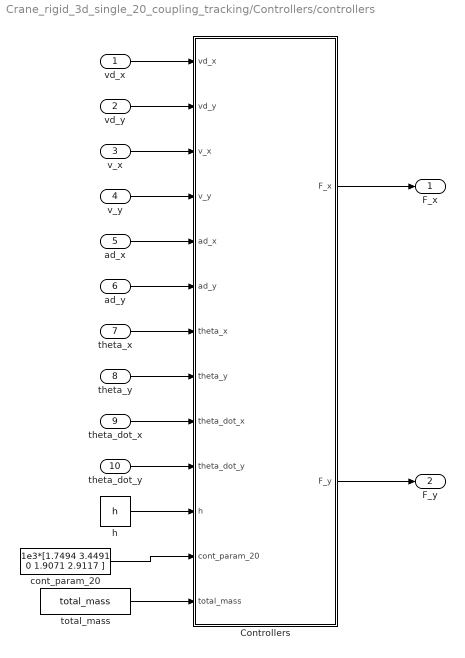
== system Crane_rigid_3d_single_20_coupling_tracking/Controllers/controllers ==
  vd_x : Inport
  vd_y : Inport  Port=2
  v_x : Inport  Port=3
  v_y : Inport  Port=4
  ad_x : Inport  Port=5
  ad_y : Inport  Port=6
  theta_x : Inport  Port=7
  theta_y : Inport  Port=8
  theta_dot_x : Inport  Port=9
  theta_dot_y : Inport  Port=10
  Controllers : MATLAB Function  TreatAsAtomicUnit=on
  cont_param_20 : Constant  Value="1e3*[1.7494    3.4491         0    1.9071    2.9117 ]"
  h : Constant  Value=h
  total_mass : Constant  Value=total_mass
  F_x : Outport
  F_y : Outport  Port=2
  wires:
  Controllers/1(F_x) -> F_x/1
  Controllers/2(F_y) -> F_y/1
  v_x/1 -> Controllers/3(v_x)
  v_y/1 -> Controllers/4(v_y)
  vd_y/1 -> Controllers/2(vd_y)
  vd_x/1 -> Controllers/1(vd_x)
  ad_x/1 -> Controllers/5(ad_x)
  ad_y/1 -> Controllers/6(ad_y)
  theta_x/1 -> Controllers/7(theta_x)
  theta_y/1 -> Controllers/8(theta_y)
  theta_dot_x/1 -> Controllers/9(theta_dot_x)
  theta_dot_y/1 -> Controllers/10(theta_dot_y)
  h/1 -> Controllers/11(h)
  total_mass/1 -> Controllers/13(total_mass)
  cont_param_20/1 -> Controllers/12(cont_param_20)

== matlab function Crane_rigid_3d_single_20_coupling_tracking/Controllers/controllers/Controllers ==
  settings: updateMethod=DISCRETE
  data: vd_x input; vd_y input; v_x input; v_y input; ad_x input; ad_y input; theta_x input; theta_y input; theta_dot_x input; theta_dot_y input; h input; cont_param_20 input; total_mass input; F_x output; F_y output
function [F_x,F_y] = Control_select(vd_x,vd_y, v_x,v_y,ad_x,ad_y, theta_x, theta_y, theta_dot_x,theta_dot_y,h,cont_param_20,total_mass)
    [F_x,F_y] = control_20_coupling_tracking_3d_first(vd_x,vd_y, v_x,v_y,ad_x,ad_y, theta_x, theta_y, theta_dot_x,theta_dot_y,h,cont_param_20,total_mass);

== matlab function Crane_rigid_3d_single_20_coupling_tracking/trajectory generator/traj1_y ==
  data: t input; x_d output; v_d output; a_d output; traj_number input; sin_traj_w input; sin_traj_A input
function [x_d,v_d,a_d] = traj_gen(t,traj_number,sin_traj_w,sin_traj_A)
     [x_d,v_d,a_d] = trajectory(t,traj_number,sin_traj_w,sin_traj_A);
end

== matlab function Crane_rigid_3d_single_20_coupling_tracking/trajectory generator/traj_x ==
  data: t input; x_d output; v_d output; a_d output; traj_number input; sin_traj_w input; sin_traj_A input
function [x_d,v_d,a_d] = traj_gen(t,traj_number,sin_traj_w,sin_traj_A)
     [x_d,v_d,a_d] = trajectory(t,traj_number,sin_traj_w,sin_traj_A);
end
